simulink model "hw2_q2"  (R2022a)
settings: Solver=VariableStepDiscrete  StartTime=0.0  StopTime=100.0  FixedStep=1  MaxStep=0.01  RelTol=1e-3
settings Model: Creator=Ariike.ir  LastModifiedBy=Ariike.ir

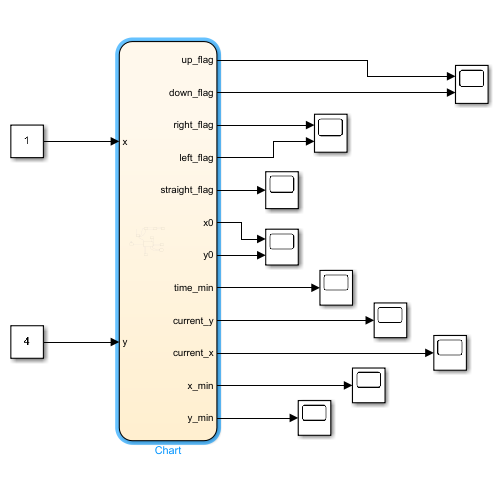
[thumbnail: Simulink's stored preview of the top-level diagram]
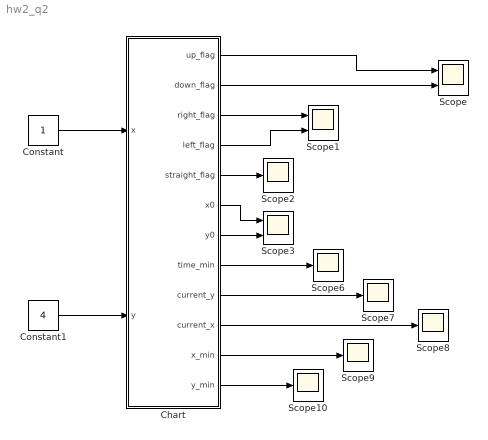
== system hw2_q2 ==
  Chart : Stateflow chart  TreatAsAtomicUnit=on
      settings: PortSchema="{\"entries\":[{\"content\":{\"sides\":[{\"content\":{\"connectorIds\":[\"In1\",\"In2\"]},\"type\":\"ConnectorPlacement.EquallySpacedRectSide\",\"uuid\":\"4977fef8-3533-48a1-ad48-3dad49daabe6\"},{\"content\":{\"connectorIds\":[\"Out1\",\"Out4\",\"Out2\",\"Out3\",\"Out5\",\"Out6\",\"Out7\",\"Out8\",\"Out9\",\"Out10\",\"Out11\",\"Out12\"],\"side\":\"RIGHT\"},\"type\":\"ConnectorPlacement.EquallySpacedRectSide\",\"uuid\":\"a781c5bc-023f-46bc-8e3e-8b3b61bfef42\"},{\"content\":{\"connectorIds\":[],\"side\":\"TOP\"},\"type\":\"ConnectorPlacement.EquallySpacedRectSide\",\"uuid\":\"71e3d3c5-e554-4944-8d32-e34412079c1f\"},{\"content\":{\"connectorIds\":[],\"side\":\"BOTTOM\"},\"type\":\"ConnectorPlacement.EquallySpacedRectSide\",\"uuid\":\"87705b30-d985-4244-988c-99e6cb477a1f\"}]},\"type\":\"ConnectorPlacement.EquallySpacedConnector\",\"uuid\":\"5398c61a-b9c7-434d-90a9-22eaf5e9b65f\"}],\"packageUris\":[\"http://schema.mathworks.com/mf0/Connector/R2020b\"],\"version\":\"1.0\"}"
  Constant : Constant
  Constant1 : Constant  Value=4
  Scope : Scope  NumInputPorts=2
  Scope1 : Scope  NumInputPorts=2
  Scope{2,6..10} (6 alike) : Scope
  Scope3 : Scope  NumInputPorts=2
  wires:
  Constant/1 -> Chart/1(x)
  Constant1/1 -> Chart/2(y)
  Chart/1(up_flag) -> Scope/1
  Chart/4(down_flag) -> Scope/2
  Chart/2(right_flag) -> Scope1/1
  Chart/3(left_flag) -> Scope1/2
  Chart/5(straight_flag) -> Scope2/1
  Chart/6(x0) -> Scope3/1
  Chart/7(y0) -> Scope3/2
  Chart/8(time_min) -> Scope6/1
  Chart/9(current_y) -> Scope7/1
  Chart/12(y_min) -> Scope10/1
  Chart/11(x_min) -> Scope9/1
  Chart/10(current_x) -> Scope8/1

== stateflow chart hw2_q2/Chart ==
  state inc_x
  state inc_y
  state check
  state start
  state right
  state stop
  state straight
  state left
  state up
  state down
  inc_y -> inc_x [order 2] : {current_y = current_y + 0.1}
  inc_y -> check [order 1] : [time_min > current_x/6 + current_y/8 + sqrt((x-current_x)*(x-current_x)+(y-current_y)*(y-current_y)) / 5]{x_min = current_x, y_min = current_y,time_min = current_x/6 + current_y/8 + sqrt((x-current_x)*(x-current_x)+(y-current_y)*(y-current_y)) / 5 }
  start -> inc_x [order 1] : [current_x<x]
  check -> inc_y
  (default) -> start : {x_min = 0
      | y_min = 0
      | time_min = 100
      | current_x = 0
      | current_y = 0
      | x0 = 0
      | y0 = 0}
  inc_x -> inc_y [order 1] : [current_y<y]
  inc_x -> start [order 2] : {current_y = 0,current_x = current_x + 0.1}
  straight -> start [order 2]
  start -> stop [order 2]
  right -> stop : {x0 = x0 + 0.1}
  stop -> right [order 1] : [x_min>x0]{right_flag = 1}
  straight -> straight [order 1] : [x~=x0 && y~=y0 ]{x0 = x0 + 0.1, y0 = y0 +0.1*((y-y0)/(x-x0))}
  stop -> left [order 2] : [x_min<x0]{left_flag = 1}
  stop -> straight [order 5] : [x~=x0 && y~=y0 ]{straight_flag = 1}
  left -> stop : {x0 = x0 - 0.1}
  down -> stop : {y0=y0-0.1}
  stop -> down [order 3] : [y_min<y0]{down_flag = 1}
  up -> stop : {y0=y0+0.1}
  stop -> up [order 4] : [y_min>y0]{up_flag = 1}
  data: x input; y input; up_flag output; right_flag output; left_flag output; down_flag output; straight_flag output; x0 output; y0 output; time_min output; current_y output; current_x output; x_min output; y_min output
